simulink model "solar"  (R2022b)
settings: Solver=FixedStepDiscrete  StartTime=0.0  StopTime=inf  FixedStep=1  RelTol=1e-3
settings Model: ExtModeTrigDuration=2  Creator=Dell  LastModifiedBy=Dell
settings OptimizationCC: DefaultParameterBehavior=Inlined  UseDivisionForNetSlopeComputation=on  GainParamInheritBuiltInType=on  UseFloatMulNetSlope=on  InlineInvariantSignals=on  PassReuseOutputArgsAs=Individual arguments  ZeroExternalMemoryAtStartup=off  ZeroInternalMemoryAtStartup=off  NoFixptDivByZeroProtection=on  EfficientFloat2IntCast=on  LifeSpan=1  MaxStackSize=64  OptimizeBlockOrder=speed  DifferentSizesBufferReuse=on  EfficientTunableParamExpr=on
settings DebuggingCC: ParameterTunabilityLossMsg=error
settings HardwareCC: ProdBitPerInt=16  ProdBitPerPointer=16  ProdBitPerSizeT=16  ProdBitPerPtrDiffT=16  ProdLargestAtomicFloat=None  ProdWordSize=8  ProdLongLongMode=on  ProdHWDeviceType=Atmel->AVR
settings SFSimCC: MATLABDynamicMemAlloc=off
settings RTWCC: Description=Embedded Coder  SystemTargetFile=ert.tlc  HardwareBoard=Arduino Uno  TLCOptions=-aInlineSetEventsForThisBaseRateFcn=TLC_FALSE -aSuppressMultiTaskScheduler=TLC_FALSE -aRateBasedStepFcn=1  TemplateMakefile=ert_default_tmf  Toolchain=Arduino AVR  BuildConfiguration=Faster Runs
settings CodeAppCC: ForceParamTrailComments=on  IgnoreCustomStorageClasses=off  OperatorAnnotations=on  SimulinkDataObjDesc=on  SFDataObjDesc=on  CustomSymbolStrGlobalVar=rt$N$M  CustomSymbolStrType=$N$M  CustomSymbolStrFcn=$N$M$F  CustomSymbolStrMacro=$N$M  InsertBlockDesc=on
settings ERTTargetCC: IncludeMdlTerminateFcn=off  CombineSignalStateStructs=on  SupportAbsoluteTime=off  SupportComplex=off  SupportNonInlinedSFcns=on  ExtModeTransport=3  ExtModeStaticAlloc=on  ExtModeAutomaticAllocSize=off  ExtModeStaticAllocSize=250  ExtModeMexFile=ext_xcp  ExtModeIntrfLevel=Level2 - Open  InlinedParameterPlacement=NonHierarchical  ERTFilePackagingFormat=CompactWithDataFile

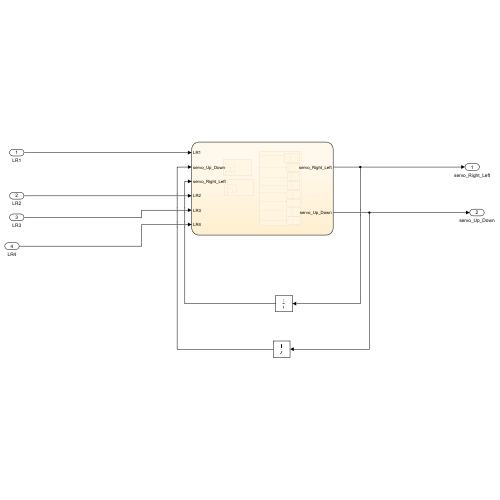
[thumbnail: Simulink's stored preview of the top-level diagram]
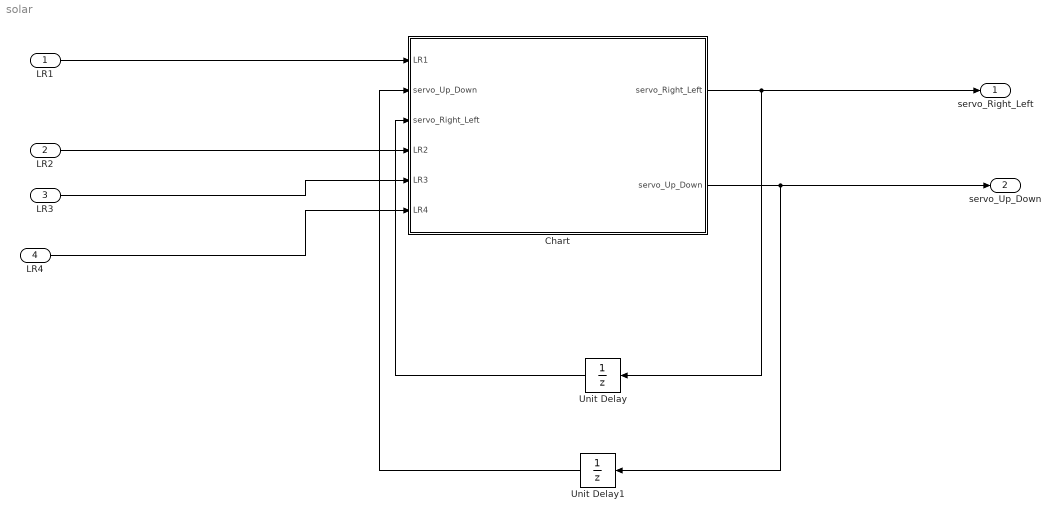
== system solar ==
  LR1 : Inport
  LR2 : Inport  Port=2
  LR3 : Inport  Port=3
  LR4 : Inport  Port=4
  Chart : Stateflow chart  TreatAsAtomicUnit=on
  Unit Delay : UnitDelay  SampleTime=-1  HasFrameUpgradeWarning=on
  Unit Delay1 : UnitDelay  SampleTime=-1  HasFrameUpgradeWarning=on
  servo_Right_Left : Outport
  servo_Up_Down : Outport  Port=2
  wires:
  LR2/1 -> Chart/4(LR2)
  LR3/1 -> Chart/5(LR3)
  LR4/1 -> Chart/6(LR4)
  Unit Delay/1 -> Chart/3("servo_Right_Left ")
  Unit Delay1/1 -> Chart/2("servo_Up_Down ")
  LR1/1 -> Chart/1(LR1)
  Chart/1(servo_Right_Left) -> servo_Right_Left/1, Unit Delay/1
  Chart/2(servo_Up_Down) -> servo_Up_Down/1, Unit Delay1/1

== stateflow chart solar/Chart ==
  state mode
    state mode_up
      (default) -> (junction 205) : {Servo_Angle(0);}
      (junction 205) -> (junction 204) : {Servo_Angle_up(90);}
    state mode_down
      (default) -> (junction 173) : {Servo_Angle(0);}
      (junction 173) -> (junction 198) : {Servo_Angle_up(-90);}
    state mode_Right
      (default) -> (junction 209) : {Servo_Angle(90);}
      (junction 209) -> (junction 208) : {Servo_Angle_up(0);}
    state mode_Left
      (default) -> (junction 213) : {Servo_Angle(-90);}
      (junction 213) -> (junction 212) : {Servo_Angle_up(0);}
    state mode_Right_Up
      (default) -> (junction 218) : {Servo_Angle(45);}
      (junction 218) -> (junction 217) : {Servo_Angle_up(45);}
    state mode_Right_Down
      (default) -> (junction 222) : {Servo_Angle(45);}
      (junction 222) -> (junction 221) : {Servo_Angle_up(-45);}
    state mode_Left_Down
      (default) -> (junction 228) : {Servo_Angle(-45);}
      (junction 228) -> (junction 227) : {Servo_Angle_up(-45);}
    state mode_Left_Up
      (default) -> (junction 232) : {Servo_Angle(-45);}
      (junction 232) -> (junction 231) : {Servo_Angle_up(45);}
    (default) -> mode_up
    mode -> mode_up [order 3] : [((LR1+LR2 )/2 >(LR3+LR4)/2) &&((LR1+LR4)/2 == (LR2+LR3)/2)]
    mode -> mode_down [order 2] : [((LR1+LR2 )/2 <(LR3+LR4)/2) &&((LR1+LR4)/2 == (LR2+LR3)/2)]
    mode -> mode_Right [order 8] : [((LR1+LR2 )/2 == (LR3+LR4)/2) &&((LR1+LR4)/2 < (LR2+LR3)/2)]
    mode -> mode_Left [order 7] : [((LR1+LR2 )/2 == (LR3+LR4)/2) &&((LR1+LR4)/2 > (LR2+LR3)/2)]
    mode -> mode_Right_Up [order 6] : [((LR1+LR2 )/2 >(LR3+LR4)/2) &&((LR1+LR4)/2 < (LR2+LR3)/2)]
    mode -> mode_Right_Down [order 5] : [((LR1+LR2 )/2  < (LR3+LR4)/2) &&((LR1+LR4)/2 < (LR2+LR3)/2)]
    mode -> mode_Left_Down [order 4] : [((LR1+LR2 )/2  < (LR3+LR4)/2) &&((LR1+LR4)/2 > (LR2+LR3)/2)]
    mode -> mode_Left_Up [order 1] : [((LR1+LR2 )/2 >(LR3+LR4)/2) &&((LR1+LR4)/2 > (LR2+LR3)/2)]
  state Servo_Angle_up(angle) [function]
    (default) -> (junction 181)
    (junction 181) -> (junction 184)
    (junction 184) -> (junction 186) [order 1] : [(servo_Up_Down >angle) && (servo_Up_Down~=angle)]
    (junction 184) -> (junction 175) [order 2]
    (junction 186) -> (junction 190) : {servo_Up_Down = servo_Up_Down - 1;}
    (junction 175) -> (junction 189) [order 1] : [(servo_Up_Down <angle) && (servo_Up_Down~=angle) ]
    (junction 175) -> (junction 191) [order 2]
    (junction 189) -> (junction 192) : {servo_Up_Down = servo_Up_Down + 1;}
    (junction 192) -> (junction 191)
    (junction 190) -> (junction 192)
    (junction 191) -> (junction 180)
  state Servo_Angle(angle) [function]
    (default) -> (junction 150)
    (junction 150) -> (junction 164)
    (junction 164) -> (junction 165) [order 1] : [(servo_Right_Left >angle) && (servo_Right_Left~=angle) ]
    (junction 164) -> (junction 166) [order 2]
    (junction 165) -> (junction 170) : {servo_Right_Left = servo_Right_Left - 1;}
    (junction 166) -> (junction 167) [order 1] : [(servo_Right_Left <angle) && (servo_Right_Left~=angle) ]
    (junction 166) -> (junction 168) [order 2]
    (junction 167) -> (junction 169) : {servo_Right_Left = servo_Right_Left + 1;}
    (junction 169) -> (junction 168)
    (junction 170) -> (junction 169)
    (junction 168) -> (junction 171)
  data: angle function_input; angle function_input; LR1 input; servo_Up_Down input; servo_Right_Left input; LR2 input; LR3 input; LR4 input; servo_Right_Left output; servo_Up_Down output
